simulink model "inverted_pendulum_linear_model_v2"  (R2018b)
settings: Solver=VariableStepAuto  StartTime=0.0  StopTime=10.0  RelTol=1e-3
values from neighbouring files (symbols this model uses):
  K = K_LQR .* 0    [main.m]
undefined symbols (not defined in the file or in its folder): A, B, C, D
settings Model: Creator=jordan  LastModifiedBy=jordan

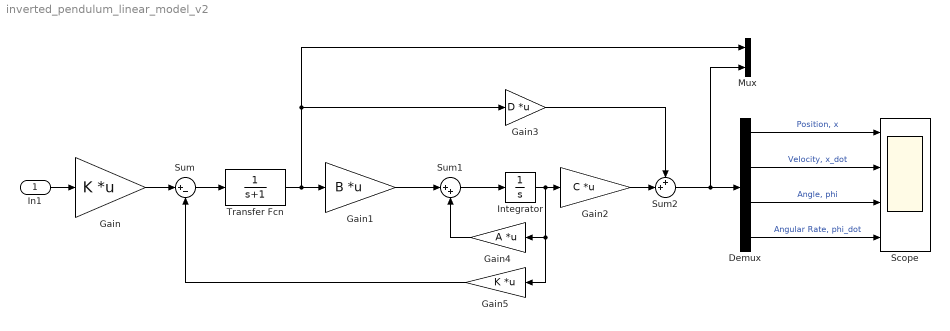
== system inverted_pendulum_linear_model_v2 ==
  In1 : Inport
  Demux : Demux
  Gain : Gain  Gain=K  Multiplication=Matrix(K*u)
  Gain1 : Gain  Gain=B  Multiplication=Matrix(K*u)
  Gain2 : Gain  Gain=C  Multiplication=Matrix(K*u)
  Gain3 : Gain  Gain=D  Multiplication=Matrix(K*u)
  Gain4 : Gain  Gain=A  Multiplication=Matrix(K*u)
  Gain5 : Gain  Gain=K  Multiplication=Matrix(K*u)
  Integrator : Integrator
  Mux : Mux  Inputs=2
  Scope : Scope  NumInputPorts=4
  Sum : Sum  Inputs=|+-
  Sum1 : Sum  Inputs=|++
  Sum2 : Sum  Inputs=++|
  Transfer Fcn : TransferFcn  Denominator=[1 1]
  wires:
  In1/1 -> Gain/1
  Sum/1 -> Transfer Fcn/1
  Gain/1 -> Sum/1
  Transfer Fcn/1 -> Mux/1, Gain3/1, Gain1/1
  Gain1/1 -> Sum1/1
  Sum1/1 -> Integrator/1
  Gain2/1 -> Sum2/2
  Gain3/1 -> Sum2/1
  Sum2/1 -> Mux/2, Demux/1
  Demux/1 -> Scope/1  "Position, x"
  Demux/3 -> Scope/3  "Angle, phi"
  Demux/2 -> Scope/2  "Velocity, x_dot"
  Demux/4 -> Scope/4  "Angular Rate, phi_dot"
  Integrator/1 -> Gain5/1, Gain4/1, Gain2/1
  Gain4/1 -> Sum1/2
  Gain5/1 -> Sum/2
